simulink model "Controllo_H_Infinito"  (R2023b)
settings: Solver=VariableStepAuto  StartTime=0.0  StopTime=50  RelTol=1e-3
undefined symbols (not defined in the file): A, Ar, B, Br, C, Cr, D, Dr, Tc
libraries: simulink x1
settings Model: Creator=emman  LastModifiedBy=emman

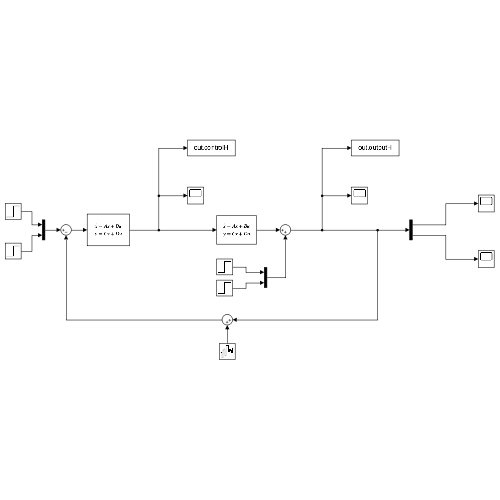
[thumbnail: Simulink's stored preview of the top-level diagram]
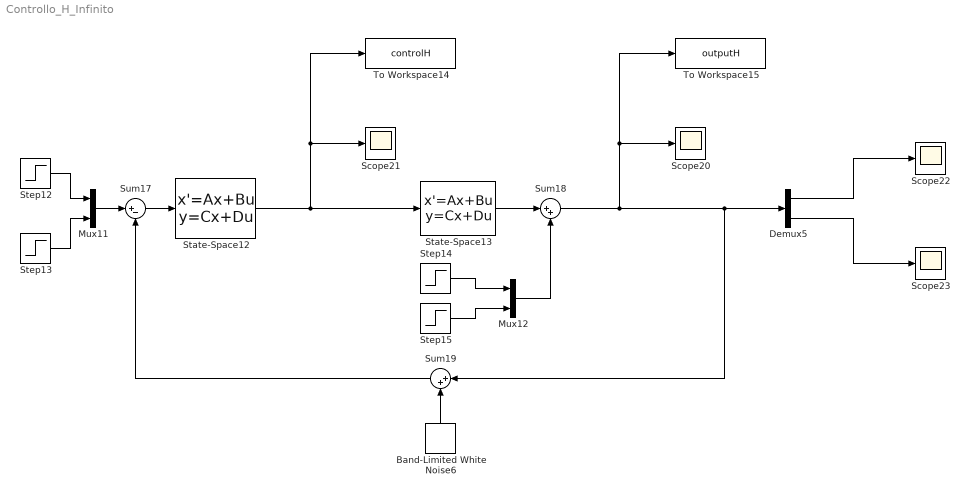
== system Controllo_H_Infinito ==
  Band-Limited White Noise6 : simulink/Sources/Band-Limited White Noise  Cov=NoisePower  Ts=Tc  seed=[23341]
  Demux5 : Demux  Outputs=2
  Mux11 : Mux  Inputs=2
  Mux12 : Mux  Inputs=2
  Scope{20..23} (4 alike) : Scope
  State-Space12 : StateSpace  A=Ar  B=Br  C=Cr  D=Dr  InitialCondition=0
  State-Space13 : StateSpace  A=A  B=B  C=C  D=D  InitialCondition=0
  Step12 : Step  Time=0  After=2  SampleTime=0
  Step13 : Step  Time=0  After=2.5  SampleTime=0
  Step14 : Step  Time=0  After=0.5  SampleTime=0
  Step15 : Step  Time=0  After=0.5  SampleTime=0
  Sum17 : Sum  Inputs=|+-
  Sum18 : Sum  Inputs=|++
  Sum19 : Sum  Inputs=|++
  To Workspace14 : ToWorkspace  VariableName=controlH  SaveFormat=Structure With Time  SampleTime=-1
  To Workspace15 : ToWorkspace  VariableName=outputH  SaveFormat=Structure With Time  SampleTime=-1
  wires:
  Step13/1 -> Mux11/2
  State-Space12/1 -> State-Space13/1, Scope21/1, To Workspace14/1
  Step15/1 -> Mux12/2
  Sum19/1 -> Sum17/2
  Demux5/1 -> Scope22/1
  Mux11/1 -> Sum17/1
  Band-Limited White Noise6/1 -> Sum19/2
  Mux12/1 -> Sum18/2
  State-Space13/1 -> Sum18/1
  Step14/1 -> Mux12/1
  Sum17/1 -> State-Space12/1
  Sum18/1 -> Sum19/1, Demux5/1, Scope20/1, To Workspace15/1
  Demux5/2 -> Scope23/1
  Step12/1 -> Mux11/1
